simulink model "aircraft"  (R2018a)
settings: Solver=VariableStepAuto  StartTime=0.0  StopTime=100  RelTol=1e-3
InitFcn:
  | P = 0;
settings Model: Creator=mark  LastModifiedBy=mark

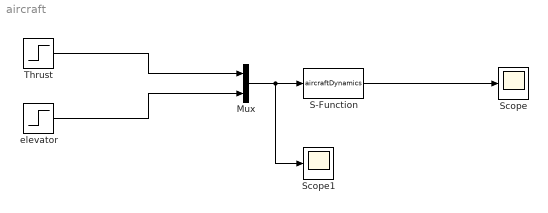
== system aircraft ==
  Mux : Mux  Inputs=2
  S-Function : S-Function  FunctionName=aircraftDynamics  Parameters=P  SFunctionDeploymentMode=off  EnableBusSupport=off
  Scope : Scope
  Scope1 : Scope
  Thrust : Step  Time=0.1  After=7  SampleTime=0
  elevator : Step  Time=10  After=0  SampleTime=0
  wires:
  Thrust/1 -> Mux/1
  elevator/1 -> Mux/2
  Mux/1 -> Scope1/1, S-Function/1
  S-Function/1 -> Scope/1
